simulink model "Three_phase_bridge_LCR"  (Simulink 6.1)
settings: Solver=ode23tb  StartTime=0.0  StopTime=0.1499  MaxStep=1e-4  RelTol=1e-3  AbsTol=.01
libraries: powerlib x14
settings Model: LastModifiedBy=ThinkPad
settings DebuggingCC: SolverPrmCheckMsg=warning

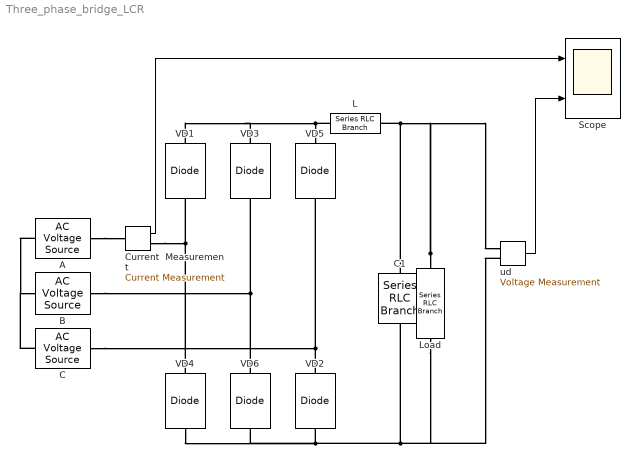
== system Three_phase_bridge_LCR ==
  A : powerlib/Electrical Sources/AC Voltage Source  Amplitude=100  Phase=30  Frequency=50  SampleTime=0  Measurements=None
  B : powerlib/Electrical Sources/AC Voltage Source  Amplitude=100  Phase=-90  Frequency=50  SampleTime=0  Measurements=None
  C : powerlib/Electrical Sources/AC Voltage Source  Amplitude=100  Phase=-210  Frequency=50  SampleTime=0  Measurements=None
  C1 : powerlib/Elements/Series RLC Branch  Orientation=up  PhysicalDomain=powersysdomain  SubClassName=unknown  LeftPortType=p1  RightPortType=p1  LConnTagsString=__new0  RConnTagsString=__new0  Resistance=0  Inductance=0  Capacitance=0.001  Measurements=None
  Current  Measurement : powerlib/Measurements/Current Measurement  PhasorSimulation=off  OutputType=Complex  PSBequivalent=0
  L : powerlib/Elements/Series RLC Branch  Orientation=left  PhysicalDomain=powersysdomain  SubClassName=unknown  LeftPortType=p1  RightPortType=p1  LConnTagsString=__new0  RConnTagsString=__new0  Resistance=0  Inductance=0.001  Capacitance=inf  Measurements=None
  Load : powerlib/Elements/Series RLC Branch  Orientation=down  PhysicalDomain=powersysdomain  SubClassName=unknown  LeftPortType=p1  RightPortType=p1  LConnTagsString=__new0  RConnTagsString=__new0  Resistance=20  Inductance=0  Capacitance=inf  Measurements=None
  Scope : Scope  NumInputPorts=2
      settings: TickLabels=on  TimeRange=0.05  YMin=-20~0  YMax=20~200  Decimation=5  SampleInput=on  SampleTime=1e-4
  VD{1..6} (6 alike) : powerlib/Power Electronics/Diode  Orientation=up  Ron=0.001  Lon=0  Vf=0.8  IC=0  Rs=500  Cs=250e-9  Measurements=off
  ud : powerlib/Measurements/Voltage Measurement  PhasorSimulation=off  OutputType=Complex  PSBequivalent=0
  wires:
  ud/1 -> Scope/2
  Current  Measurement/1 -> Scope/1
  connections:
  C1/RConn1 -- Load/LConn1 -- ud/LConn1 -- L/LConn1
  VD1/RConn1 -- VD3/RConn1 -- VD5/RConn1 -- L/RConn1
  A/LConn1 -- C/LConn1 -- B/LConn1
  VD4/RConn1 -- VD1/LConn1 -- Current  Measurement/RConn1
  ud/LConn2 -- Load/RConn1 -- VD4/LConn1 -- VD6/LConn1 -- VD2/LConn1 -- C1/LConn1
  C/RConn1 -- VD2/RConn1 -- VD5/LConn1
  B/RConn1 -- VD6/RConn1 -- VD3/LConn1
  A/RConn1 -- Current  Measurement/LConn1
